simulink library "rotations_Lib"  (R2018b)
settings: Solver=VariableStepAuto  StartTime=0.0  StopTime=10.0  RelTol=1e-3
settings Model: Creator=IvanMachuca  LastModifiedBy=devantormey

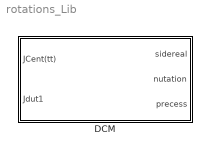
== system rotations_Lib ==
  "DCM " : Subsystem

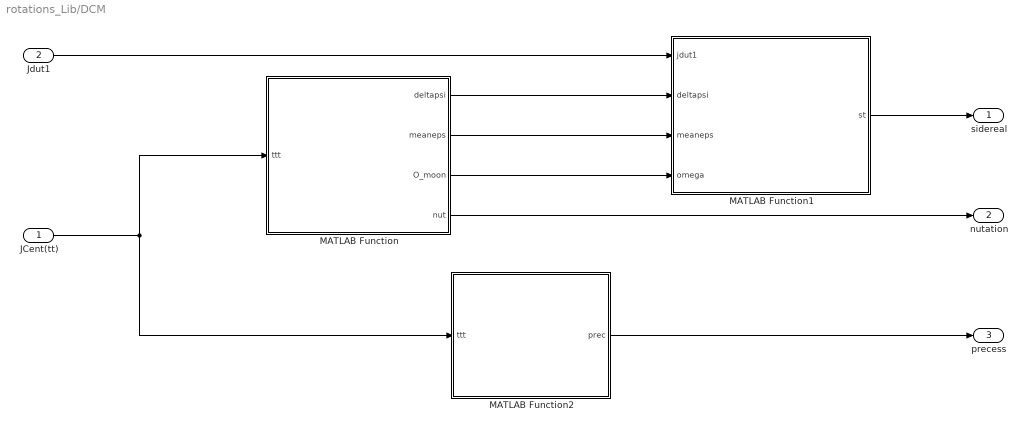
== system rotations_Lib/DCM  ==
  "JCent(tt) " : Inport
  Jdut1 : Inport  Port=2
  MATLAB Function : MATLAB Function  TreatAsAtomicUnit=on
  MATLAB Function1 : MATLAB Function  TreatAsAtomicUnit=on
  MATLAB Function2 : MATLAB Function  TreatAsAtomicUnit=on
  "sidereal " : Outport
  "nutation " : Outport  Port=2
  "precess " : Outport  Port=3
  wires:
  MATLAB Function/1(deltapsi) -> MATLAB Function1/2(deltapsi)
  MATLAB Function2/1(prec) -> "precess "/1
  "JCent(tt) "/1 -> MATLAB Function2/1(ttt), MATLAB Function/1(ttt)
  Jdut1/1 -> MATLAB Function1/1(jdut1)
  MATLAB Function/4(nut) -> "nutation "/1
  MATLAB Function1/1(st) -> "sidereal "/1
  MATLAB Function/2(meaneps) -> MATLAB Function1/3(meaneps)
  MATLAB Function/3(O_moon) -> MATLAB Function1/4(omega)

== matlab function rotations_Lib/DCM /MATLAB Function2 ==
  data: ttt input; prec output
%Author-Ivan Machuca
%Date - 1/31/19

%This function inputs ttt and outputs the precession angles and precession
%transformation matrix. 

function prec  = precess_funct(ttt)
%ttt is the julian century in teresterial time 
ttt2=ttt.^2; 
ttt3=ttt.^3;
deg_rad=pi/(180.0*3600); %changing degrees to radians Not sure why multiplying by 3600

%Calculting the iau 76 precession angles in radians
 psia = deg_rad*(5038.7784*ttt - 1.07259*ttt2 - 0.001147*ttt3); 
 wa   = deg_rad*(84381.448+ 0.05127*ttt2 - 0.007726*ttt3);
 ea   = deg_rad*(84381.448 -46.8150*ttt - 0.00059*ttt2 + 0.001813*ttt3);
 xa   = deg_rad*(10.5526*ttt - 2.38064*ttt2 - 0.001125*ttt3);
 
 
 
 zeta = deg_rad*(2306.2181*ttt + 0.30188*ttt2 + 0.017998*ttt3);
 theta= deg_rad*(2004.3109*ttt - 0.42665*ttt2 - 0.041833*ttt3);
 z    = deg_rad*(2306.2181*ttt + 1.09468*ttt2 + 0.018203*ttt3);

%Getting the angles 
coszeta  = cos(zeta);
sinzeta  = sin(zeta);
costheta = cos(theta);
sintheta = sin(theta);
cosz     = cos(z);
sinz     = sin(z);

%Calculating the precession rotation matrix for transformation
 prec(1,1) =  coszeta * costheta * cosz - sinzeta * sinz;
 prec(1,2) =  coszeta * costheta * sinz + sinzeta * cosz;
 prec(1,3) =  coszeta * sintheta;
 prec(2,1) = -sinzeta * costheta * cosz - coszeta * sinz;
 prec(2,2) = -sinzeta * costheta * sinz + coszeta * cosz;
 prec(2,3) = -sinzeta * sintheta;
 prec(3,1) = -sintheta * cosz;
 prec(3,2) = -sintheta * sinz;
 prec(3,3) =  costheta;
 
 

end

== matlab function rotations_Lib/DCM /MATLAB Function ==
  data: ttt input; deltapsi output; meaneps output; O_moon output; nut output
%Author Kate Williams
%Date 1/24/2019

%Last edit by Kate Williams 2/14/2019, changed method of final matrix to use rot1,rot3
%terms
%conversions
function [deltapsi, meaneps,O_moon,nut] = nutation(ttt)
        %OUTPUT ANGLES IN RADIANTS
        deg2rad = pi/180.0; %deg to rad
        rad2deg = 1/deg2rad;
        asec2rad = 1/3600*deg2rad;
        ttt2= ttt*ttt; %ttt is julian century in tt time frame
        ttt3= ttt2*ttt;
        
        %mean obliquity of the ecliptic in rads
        meaneps = deg2rad * ( 23.439291 ...
                        - 0.0130042 * ttt ...
                        - 1.64e-7 * ttt2 ...
                        + 5.04e-7 * ttt3);
                % ---- iau 1980 theory
% Largest Nutation coefficents (out of 106)                    
        nc = [ ...
            1   0   0   0   0   1   -171996 -174.2  92025   8.9
            9   0   0   2   -2  2   -13187  -1.6    5736    -3.1
            31  0   0   2   0   2   -2274   -0.2    977     -0.5
            2   0   0   0   0   2   2062    0.2     -895    0.5
            10  0   1   0  	0   0   1426    -3.4    54      -0.1
            32  1   0   0   0   0   712     0.1     -7      0.0
            11  0   1   2   -2  2   -517    1.2     224     -0.6
            33  0   0   2   0   1   -386    -0.4    200     0.0
            34  1   0   2   0   2   -301    0.0     129     -0.1
            12  0   -1  2   -2  2   217     -0.5    -95     0.3
            35  1   0   0   -2  0   -158    0.0     -1      0.0
            13  0   0   2   -2  1   129     0.1     -70     0.0 
            36  -1  0   2   0   2   123     0.0     -53     0.0 
            38  1   0   0   0   1   63      0.1     -33     0.0
            37  0   0   0   2   0   63      0.0     -2      0.0
            40  -1  0   2   2   2   -59     0.0     26      0.0
            39  -1  0   0   0   1   -58     -0.1    32      0.0
            41  1   0   2   0   1   -51     0.0     27      0.0
            14  2   0   0   -2  0   48      0.0     1       0.0
            3   -2  0   2   0   1   46      0.0     -24     0.0
            42  0   0   2   2   2   -38     0.0     16      0.0
            45  2   0   2   0   2   -31     0.0     13      0.0
            43  2   0   0   0   0   29      0.0     -1      0.0
            44  1   0   2   -2  2   29      0.0     -12     0.0
            46  0   0   2   0   0   26      0.0     -1      0.0
            15  0   0   2   -2  0   -22     0.0     0       0.0
            47  -1  0   2   0   1   21      0.0     -10     0.0
            16  0   2   0   0   0   17      -0.1    0       0.0
            18  0   2   2   -2  2   -16     0.1     7       0.0
            48  -1  0   0   2   1   16      0.0     -8      0.0 ...
            ];
        
        M_moon	=   deg2rad * ( 134.96298139+(1325 * 360 + 198.8673981) * ttt ...
                      	+ 0.0086972 * ttt2 + 1.78e-5 * ttt3);
               
        M_sun	=   deg2rad * ( 357.52772333 + (99 * 360 + 359.0503400) * ttt ...
                        - 0.0001603 * ttt2 - 3.3e-6 * ttt3);

        U_moon	=   deg2rad * ( 93.27191028 + (1342 * 360 + 82.0175381) * ttt ...
                        - 0.0036825 * ttt2 + 3.1e-6 * ttt3);

        D_sun	=   deg2rad * ( 297.85036306 + (1236 * 360 + 307.1114800) * ttt ...
                        - 0.0019142 * ttt^2 + 5.3e-6 *ttt^3);

        O_moon	=   deg2rad * ( 125.04452222 - (5 * 360 + 134.1362608) * ttt ...
                        + 0.0020708 * ttt^2 + 2.2e-6 * ttt^3);       
            
        % ---- ANGLES of nutation from equ 3-82 of vallado 
        M_moon    = rem( M_moon,360.0  )     * deg2rad; % rad %moon
        M_sun   = rem( M_sun,360.0  )    * deg2rad;%sun
        U_moon    = rem( U_moon,360.0  )     * deg2rad;%moon
        D_sun    = rem( D_sun,360.0  )     * deg2rad;%sun
        O_moon= rem( O_moon,360.0  ) * deg2rad;%moon
        
        %find nutation in longitude and nutation in obliquity
        deltapsi= 0.0; %nutation angle in rad set initially to zero
        deltaeps= 0.0; %change in obliquity in rad
        
        for i = 1:size(nc,1)
            tempval    =   nc(i,2) * M_moon + nc(i,3) * M_sun + nc(i,4) * U_moon + nc(i,5) * D_sun + nc(i,6) * O_moon;
            deltapsi   =   0.0001 * (nc(i,7) + nc(i,8) * ttt) * sin(tempval) + deltapsi;
            deltaeps   =   0.0001 * (nc(i,9) + nc(i,10) * ttt) * cos(tempval) + deltaeps;
        end

        
        %final nutation parameters, see page 226 equ. 3-85of Vallado
        trueeps  = meaneps + deltaeps*asec2rad; %true obliquity of eclipti

        %complete nutation rotation matrix
        nut=zeros(3);
        
        rot1_meaneps=[1 0 0;0 cos(-meaneps) sin(-meaneps);0 -sin(-meaneps) cos(-meaneps)];
        rot3_deltapsi=[cos(asec2rad * deltapsi) sin(asec2rad * deltapsi) 0;-sin(asec2rad * deltapsi) cos(asec2rad * deltapsi) 0;0 0 1];
        rot1_trueeps=[1 0 0;0 cos(trueeps) sin(trueeps);0 -sin(trueeps) cos(trueeps)];
        
        nut = rot1_meaneps* rot3_deltapsi* rot1_trueeps;   
        
         %testing THis must be kept. 
        deltapsi = deltapsi*asec2rad; 
        deltaeps = deltaeps*asec2rad;
end

== matlab function rotations_Lib/DCM /MATLAB Function1 ==
  data: jdut1 input; st output; deltapsi input; meaneps input; omega input
function st  = sidereal(jdut1,deltapsi,meaneps,omega)

%SUMMARY: Tthis function calulates the transformation matrix that accounts for the
%    effects of sidereal time.
% inputs          description                    range / units
%    jdut1       - julian centuries of ut1        days
%    deltapsi    - nutation angle                 rad
%    meaneps     - mean obliquity of the ecliptic rad
%    omega       - long of asc node of moon       rad
%    lod         - length of day                  sec
%    eqeterms    - terms for ast calculation      0,2
%
%  outputs       :
%    st          - transformation matrix for pef - tod
%    stdot       - transformation matrix for pef - tod rate
%  locals        :
%    gmst        - mean greenwich sidereal time   0 to 2pi rad
%    ast         - apparent gmst                   0 to 2pi rad
%    hr          - hour                           hr
%    min         - minutes                        min
%    sec         - seconds                        sec
%    temp        - temporary vector
%    tempval     - temporary variable

% Constants
twopi      = 2.0*pi;
deg2rad    = pi/180.0;
lod = .0015563;

% ------------------------  Find GMST   ------------------
% ////////////////////////////////////////////////////////

tut1= ( jdut1 - 2451545.0 ) / 36525.0;

temp = - 6.2e-6 * tut1 * tut1 * tut1 + 0.093104 * tut1 * tut1  ...
               + (876600.0 * 3600.0 + 8640184.812866) * tut1 +...
               67310.54841; %Vallado Online Code

% 360/86400 = 1/240, to deg, to rad
temp = mod(temp*deg2rad/240.0,twopi);

% ------------------------ check quadrants -----------------
        if ( temp < 0.0 )
            temp = temp + twopi;
        end

gmst = temp;

% ////////////////////////////////////////////////////////
% ----------------------------------------------------------


% ------------------------ Find Mean AST ------------------
% ////////////////////////////////////////////////////////

if (jdut1 > 2450449.5 )
    ast= gmst + deltapsi* cos(meaneps) ...
        + 0.00264*pi /(3600*180)*sin(omega) ...
        + 0.000063*pi /(3600*180)*sin(2.0 *omega);
else
    ast= gmst + deltapsi* cos(meaneps);
end

ast        = mod(ast, 2.0*pi);
thetasa    = 7.29211514670698e-05 * (1.0  - lod/86400.0 );
omegaearth = thetasa;

% ////////////////////////////////////////////////////////
% ----------------------------------------------------------

% -------------- Calculate the Rotation Matrices -------------
% /////////////////////////////////////////////////////////////
fprintf(1,'st gmst %11.8f ast %11.8f ome  %11.8f \n', gmst*180/pi, ast*180/pi, omegaearth*180/pi );

        st(1,1) =  cos(ast);
        st(1,2) = -sin(ast);
        st(1,3) =  0.0;
        st(2,1) =  sin(ast);
        st(2,2) =  cos(ast);
        st(2,3) =  0.0;
        st(3,1) =  0.0;
        st(3,2) =  0.0;
        st(3,3) =  1.0;

% compute sidereal time rate matrix
        stdot(1,1) = -omegaearth * sin(ast);
        stdot(1,2) = -omegaearth * cos(ast);
        stdot(1,3) =  0.0;
        stdot(2,1) =  omegaearth * cos(ast);
        stdot(2,2) = -omegaearth * sin(ast);
        stdot(2,3) =  0.0;
        stdot(3,1) =  0.0;
        stdot(3,2) =  0.0;
        stdot(3,3) =  0.0;
        
% ////////////////////////////////////////////////////////
% ----------------------------------------------------------

end
